simulink model "controlador_sugeno_obstaculos_velocidad"  (R2019a)
settings: Solver=FixedStepDiscrete  StartTime=0.0  StopTime=200  FixedStep=0.1  RelTol=1e-3
values from neighbouring files (symbols this model uses):
  arround_th = 0.01    [sugeno_obstaculos_velocidad.m]
  gain = 0.8    [sugeno_obstaculos_velocidad.m]
  offset_0 = -0.2    [sugeno_obstaculos_velocidad.m]
  offset_1 = -0.22    [sugeno_obstaculos_velocidad.m]
  offset_2 = -0.18    [sugeno_obstaculos_velocidad.m]
  offset_obs1 = 1.82    [sugeno_obstaculos_velocidad.m]
  offset_obs2 = -0.06    [sugeno_obstaculos_velocidad.m]
  saturation1_high = 1.27    [sugeno_obstaculos_velocidad.m]
  saturation1_high_lineal = 1.11    [sugeno_obstaculos_velocidad.m]
  saturation1_low = -1.39    [sugeno_obstaculos_velocidad.m]
  saturation1_low_lineal = -1.38    [sugeno_obstaculos_velocidad.m]
  saturation2_high = 4.53    [sugeno_obstaculos_velocidad.m]
  saturation2_high_lineal = 4.25    [sugeno_obstaculos_velocidad.m]
  saturation2_low = -4.47    [sugeno_obstaculos_velocidad.m]
  saturation2_low_lineal = -4.15    [sugeno_obstaculos_velocidad.m]
  saturation3_high = 3.31    [sugeno_obstaculos_velocidad.m]
  saturation3_high_lineal = 3.30    (= 3.3)    [sugeno_obstaculos_velocidad.m]
  saturation3_low = -2.01    [sugeno_obstaculos_velocidad.m]
  saturation3_low_lineal = -2    [sugeno_obstaculos_velocidad.m]
  saturation4_high = 2.37    [sugeno_obstaculos_velocidad.m]
  saturation4_high_lineal = 2.31    [sugeno_obstaculos_velocidad.m]
  saturation4_low = -5    [sugeno_obstaculos_velocidad.m]
  saturation4_low_lineal = -5    [sugeno_obstaculos_velocidad.m]
  saturation5_high = 4.71    [sugeno_obstaculos_velocidad.m]
  saturation5_high_lineal = 4.57    [sugeno_obstaculos_velocidad.m]
  saturation5_low = -3.57    [sugeno_obstaculos_velocidad.m]
  saturation5_low_lineal = -2.87    [sugeno_obstaculos_velocidad.m]
  Ts = 100e-3    (= 0.1)    [sugeno_obstaculos_velocidad.m]
undefined symbols (not defined in the file or in its folder): Angular, Linear
libraries: robotlib x11, fuzblock x2, robotcorelib x1
settings Model: EnablePacing=on  Creator=pizarro  LastModifiedBy=juanjosecordoba
settings DataIOCC: ReturnWorkspaceOutputs=off

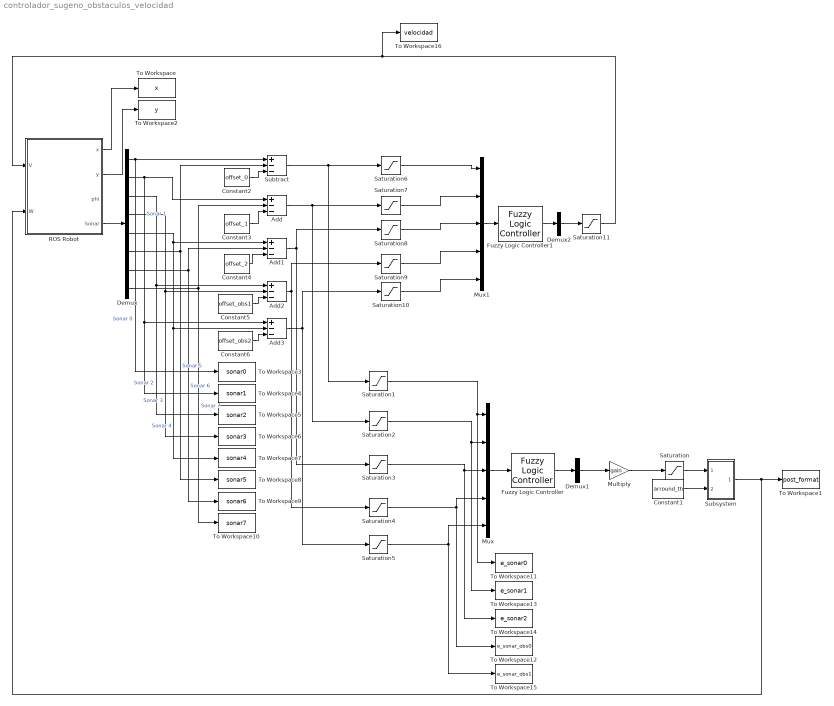
== system controlador_sugeno_obstaculos_velocidad ==
  Add{,1..3} (4 alike) : Sum  Inputs=+--
  Constant1 : Constant  Value=arround_th
  Constant2 : Constant  Value=offset_0  SampleTime=Ts
  Constant3 : Constant  Value=offset_1  SampleTime=Ts
  Constant4 : Constant  Value=offset_2  SampleTime=Ts
  Constant5 : Constant  Value=offset_obs1  SampleTime=Ts
  Constant6 : Constant  Value=offset_obs2  SampleTime=Ts
  Demux : Demux  Outputs=8
  Demux1 : Demux  Outputs=1
  Demux2 : Demux  Outputs=1
  Fuzzy Logic Controller : fuzblock/Fuzzy Logic  Controller  FIS=controller_name  OutputSampleNumber=101  DataType=double  FuzzifiedInputs=off  RuleFiringStrengths=off  RuleOutputs=off  AggregatedOutputs=off  SimulateUsing=Interpreted execution  OutOfRangeInputValueMessage=warning  NoRuleFiredMessage=warning  EmptyOutputFuzzySetMessage=warning
  Fuzzy Logic Controller1 : fuzblock/Fuzzy Logic  Controller  FIS=controller_name_lineal  OutputSampleNumber=101  DataType=double  FuzzifiedInputs=off  RuleFiringStrengths=off  RuleOutputs=off  AggregatedOutputs=off  SimulateUsing=Interpreted execution  OutOfRangeInputValueMessage=warning  NoRuleFiredMessage=warning  EmptyOutputFuzzySetMessage=warning
  Multiply : Gain  Gain=gain
  Mux : Mux  Inputs=5
  Mux1 : Mux  Inputs=5
  ROS Robot : Subsystem
  Saturation : Saturate  UpperLimit=pi  LowerLimit=-pi
  Saturation1 : Saturate  UpperLimit=saturation1_high  LowerLimit=saturation1_low
  Saturation10 : Saturate  UpperLimit=saturation5_high_lineal  LowerLimit=saturation5_low_lineal
  Saturation11 : Saturate  UpperLimit=1  LowerLimit=0
  Saturation2 : Saturate  UpperLimit=saturation2_high  LowerLimit=saturation2_low
  Saturation3 : Saturate  UpperLimit=saturation3_high  LowerLimit=saturation3_low
  Saturation4 : Saturate  UpperLimit=saturation4_high  LowerLimit=saturation4_low
  Saturation5 : Saturate  UpperLimit=saturation5_high  LowerLimit=saturation5_low
  Saturation6 : Saturate  UpperLimit=saturation1_high_lineal  LowerLimit=saturation1_low_lineal
  Saturation7 : Saturate  UpperLimit=saturation2_high_lineal  LowerLimit=saturation2_low_lineal
  Saturation8 : Saturate  UpperLimit=saturation3_high_lineal  LowerLimit=saturation3_low_lineal
  Saturation9 : Saturate  UpperLimit=saturation4_high_lineal  LowerLimit=saturation4_low_lineal
  Subsystem : Subsystem
  Subtract : Sum  Inputs=+--
  To Workspace : ToWorkspace  VariableName=x  SaveFormat=Structure With Time  SampleTime=Ts
  To Workspace1 : ToWorkspace  VariableName=post_format  SaveFormat=Structure With Time  SampleTime=Ts
  To Workspace10 : ToWorkspace  VariableName=sonar7  SaveFormat=Structure With Time  SampleTime=Ts
  To Workspace11 : ToWorkspace  VariableName=e_sonar0  SaveFormat=Structure With Time  SampleTime=Ts
  To Workspace12 : ToWorkspace  VariableName=e_sonar_obs0  SaveFormat=Structure With Time  SampleTime=Ts
  To Workspace13 : ToWorkspace  VariableName=e_sonar1  SaveFormat=Structure With Time  SampleTime=Ts
  To Workspace14 : ToWorkspace  VariableName=e_sonar2  SaveFormat=Structure With Time  SampleTime=Ts
  To Workspace15 : ToWorkspace  VariableName=e_sonar_obs1  SaveFormat=Structure With Time  SampleTime=Ts
  To Workspace16 : ToWorkspace  VariableName=velocidad  SaveFormat=Structure With Time  SampleTime=Ts
  To Workspace2 : ToWorkspace  VariableName=y  SaveFormat=Structure With Time  SampleTime=Ts
  To Workspace3 : ToWorkspace  VariableName=sonar0  SaveFormat=Structure With Time  SampleTime=Ts
  To Workspace4 : ToWorkspace  VariableName=sonar1  SaveFormat=Structure With Time  SampleTime=Ts
  To Workspace5 : ToWorkspace  VariableName=sonar2  SaveFormat=Structure With Time  SampleTime=Ts
  To Workspace6 : ToWorkspace  VariableName=sonar3  SaveFormat=Structure With Time  SampleTime=Ts
  To Workspace7 : ToWorkspace  VariableName=sonar4  SaveFormat=Structure With Time  SampleTime=Ts
  To Workspace8 : ToWorkspace  VariableName=sonar5  SaveFormat=Structure With Time  SampleTime=Ts
  To Workspace9 : ToWorkspace  VariableName=sonar6  SaveFormat=Structure With Time  SampleTime=Ts
  wires:
  ROS Robot/4(Sonar) -> Demux/1
  Fuzzy Logic Controller/1 -> Demux1/1
  Mux/1 -> Fuzzy Logic Controller/1
  Demux/1 -> Subtract/1, To Workspace3/1  "Sonar 0"
  Demux1/1 -> Multiply/1
  Saturation/1 -> Subsystem/1(value)
  Subsystem/1(Out1) -> ROS Robot/2(W), To Workspace1/1
  Constant1/1 -> Subsystem/2(arround_zero)
  Constant2/1 -> Subtract/3
  Constant3/1 -> Add/3
  Constant4/1 -> Add1/3
  Demux/2 -> Add3/1, To Workspace4/1, Add/1  "Sonar 1"
  Demux/6 -> Subtract/2, To Workspace8/1  "Sonar 5"
  Demux/5 -> Add3/2, To Workspace7/1, Add1/1  "Sonar 4"
  Demux/8 -> Add/2, To Workspace10/1  "Sonar 7"
  Demux/7 -> To Workspace9/1, Add1/2  "Sonar 6"
  Constant5/1 -> Add2/3
  Demux/3 -> To Workspace5/1, Add2/1  "Sonar 2"
  Demux/4 -> Add2/2, To Workspace6/1  "Sonar 3"
  Constant6/1 -> Add3/3
  ROS Robot/1(x) -> To Workspace/1
  ROS Robot/2(y) -> To Workspace2/1
  Subtract/1 -> Saturation6/1, Saturation1/1
  Add/1 -> Saturation7/1, Saturation2/1
  Add1/1 -> Saturation8/1, Saturation3/1
  Add2/1 -> Saturation9/1, Saturation4/1
  Add3/1 -> Saturation10/1, Saturation5/1
  Multiply/1 -> Saturation/1
  Saturation1/1 -> To Workspace11/1, Mux/1
  Saturation2/1 -> Mux/2, To Workspace13/1
  Saturation3/1 -> Mux/3, To Workspace14/1
  Saturation4/1 -> To Workspace12/1, Mux/4
  Saturation5/1 -> To Workspace15/1, Mux/5
  Saturation7/1 -> Mux1/2
  Saturation10/1 -> Mux1/5
  Saturation6/1 -> Mux1/1
  Saturation9/1 -> Mux1/4
  Saturation8/1 -> Mux1/3
  Mux1/1 -> Fuzzy Logic Controller1/1
  Fuzzy Logic Controller1/1 -> Demux2/1
  Demux2/1 -> Saturation11/1
  Saturation11/1 -> ROS Robot/1(V), To Workspace16/1

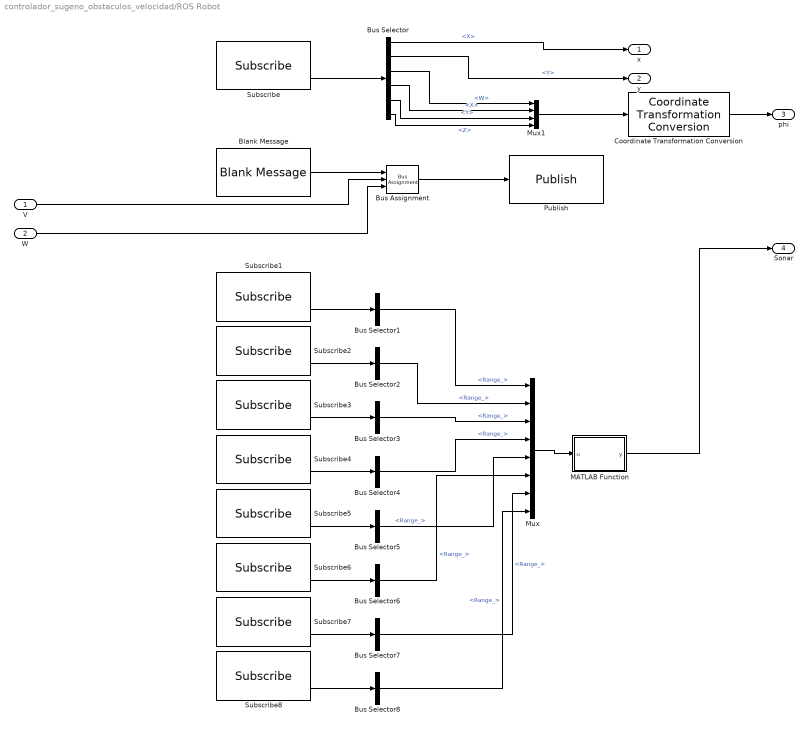
== system controlador_sugeno_obstaculos_velocidad/ROS Robot ==
  V : Inport
  W : Inport  Port=2
  Blank Message : robotlib/Blank Message  messageClass=Message  entityType=geometry_msgs/Twist  messageType=geometry_msgs/Twist  SampleTime=-1
      settings: SourceProductBaseCode=RO
  Bus Assignment : BusAssignment  AssignedSignals=Linear.X,Angular.Z
  Bus Selector : BusSelector  OutputSignals=Pose.Pose.Position.X,Pose.Pose.Position.Y,Pose.Pose.Orientation.W,Pose.Pose.Orientation.X,Pose.Pose.Orientation.Y,Pose.Pose.Orientation.Z
  Bus Selector{1..8} (8 alike) : BusSelector  OutputSignals=Range_
  Coordinate Transformation Conversion : robotcorelib/Coordinate Transformation Conversion  InputRepresentation=Quaternion  InputEulerSequence=ZYX  ShowTrVecInputPort=on  OutputRepresentation=Euler Angles  OutputEulerSequence=ZYX  ShowTrVecOutputPort=on  SimulateUsing=Interpreted execution
      settings: SourceProductBaseCode=RO
  MATLAB Function : MATLAB Function  TreatAsAtomicUnit=on
  Mux : Mux  Inputs=8
  Mux1 : Mux
  Publish : robotlib/Publish  topicSource=Select from ROS network  topic=/robot0/cmd_vel  messageType=geometry_msgs/Twist  messageQueueLength=1
      settings: SourceProductBaseCode=RO
  Subscribe : robotlib/Subscribe  topicSource=Select from ROS network  topic=/robot0/odom  messageType=nav_msgs/Odometry  sampleTime=-1  messageQueueLength=1
      settings: SourceProductBaseCode=RO
  Subscribe1 : robotlib/Subscribe  topicSource=Select from ROS network  topic=/robot0/sonar_0  messageType=sensor_msgs/Range  sampleTime=-1  messageQueueLength=1
      settings: SourceProductBaseCode=RO
  Subscribe2 : robotlib/Subscribe  topicSource=Select from ROS network  topic=/robot0/sonar_1  messageType=sensor_msgs/Range  sampleTime=-1  messageQueueLength=1
      settings: SourceProductBaseCode=RO
  Subscribe3 : robotlib/Subscribe  topicSource=Select from ROS network  topic=/robot0/sonar_2  messageType=sensor_msgs/Range  sampleTime=-1  messageQueueLength=1
      settings: SourceProductBaseCode=RO
  Subscribe4 : robotlib/Subscribe  topicSource=Select from ROS network  topic=/robot0/sonar_3  messageType=sensor_msgs/Range  sampleTime=-1  messageQueueLength=1
      settings: SourceProductBaseCode=RO
  Subscribe5 : robotlib/Subscribe  topicSource=Select from ROS network  topic=/robot0/sonar_4  messageType=sensor_msgs/Range  sampleTime=-1  messageQueueLength=1
      settings: SourceProductBaseCode=RO
  Subscribe6 : robotlib/Subscribe  topicSource=Select from ROS network  topic=/robot0/sonar_5  messageType=sensor_msgs/Range  sampleTime=-1  messageQueueLength=1
      settings: SourceProductBaseCode=RO
  Subscribe7 : robotlib/Subscribe  topicSource=Select from ROS network  topic=/robot0/sonar_6  messageType=sensor_msgs/Range  sampleTime=-1  messageQueueLength=1
      settings: SourceProductBaseCode=RO
  Subscribe8 : robotlib/Subscribe  topicSource=Select from ROS network  topic=/robot0/sonar_7  messageType=sensor_msgs/Range  sampleTime=-1  messageQueueLength=1
      settings: SourceProductBaseCode=RO
  x : Outport
  y : Outport  Port=2
  phi : Outport  Port=3
  Sonar : Outport  Port=4
  wires:
  Bus Selector/1 -> x/1  "<X>"
  Blank Message/1 -> Bus Assignment/1
  Subscribe/2 -> Bus Selector/1
  Bus Assignment/1 -> Publish/1
  Bus Selector/2 -> y/1  "<Y>"
  Subscribe1/2 -> Bus Selector1/1
  V/1 -> Bus Assignment/2
  W/1 -> Bus Assignment/3
  Subscribe2/2 -> Bus Selector2/1
  Subscribe3/2 -> Bus Selector3/1
  Subscribe5/2 -> Bus Selector5/1
  Subscribe4/2 -> Bus Selector4/1
  Subscribe6/2 -> Bus Selector6/1
  Subscribe7/2 -> Bus Selector7/1
  Bus Selector1/1 -> Mux/1  "<Range_>"
  Bus Selector2/1 -> Mux/2  "<Range_>"
  Bus Selector3/1 -> Mux/3  "<Range_>"
  Bus Selector4/1 -> Mux/4  "<Range_>"
  Bus Selector5/1 -> Mux/5  "<Range_>"
  Bus Selector6/1 -> Mux/6  "<Range_>"
  Bus Selector7/1 -> Mux/7  "<Range_>"
  Subscribe8/2 -> Bus Selector8/1
  Bus Selector8/1 -> Mux/8  "<Range_>"
  Bus Selector/3 -> Mux1/1  "<W>"
  Bus Selector/4 -> Mux1/2  "<X>"
  Bus Selector/5 -> Mux1/3  "<Y>"
  Bus Selector/6 -> Mux1/4  "<Z>"
  Mux1/1 -> Coordinate Transformation Conversion/1
  Coordinate Transformation Conversion/1 -> phi/1
  Mux/1 -> MATLAB Function/1(u)
  MATLAB Function/1(y) -> Sonar/1

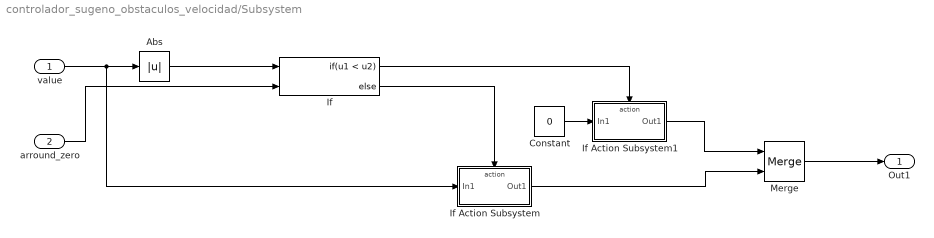
== system controlador_sugeno_obstaculos_velocidad/Subsystem ==
  value : Inport
  arround_zero : Inport  Port=2
  Abs : Abs
  Constant : Constant  Value=0  SampleTime=Ts
  If : If  NumInputs=2  IfExpression=u1 < u2
  If Action Subsystem : Subsystem  TreatAsAtomicUnit=on
  If Action Subsystem1 : Subsystem  TreatAsAtomicUnit=on
  Merge : Merge
  Out1 : Outport
  wires:
  If/1 -> If Action Subsystem1/Action
  If/2 -> If Action Subsystem/Action
  arround_zero/1 -> If/2
  If Action Subsystem1/1(Out1) -> Merge/1
  If Action Subsystem/1(Out1) -> Merge/2
  Merge/1 -> Out1/1
  value/1 -> Abs/1, If Action Subsystem/1(In1)
  Constant/1 -> If Action Subsystem1/1(In1)
  Abs/1 -> If/1

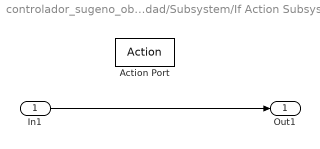
== system controlador_sugeno_obstaculos_velocidad/Subsystem/If Action Subsystem ==
  In1 : Inport
  Action Port : ActionPort  ActionPortLabel=else
  Out1 : Outport
  wires:
  In1/1 -> Out1/1

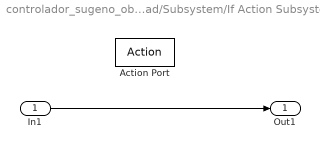
== system controlador_sugeno_obstaculos_velocidad/Subsystem/If Action Subsystem1 ==
  In1 : Inport
  Action Port : ActionPort  ActionPortLabel=if(u1 < u2)
  Out1 : Outport
  wires:
  In1/1 -> Out1/1

== matlab function controlador_sugeno_obstaculos_velocidad/ROS Robot/MATLAB Function ==
  data: u input; y output
function y = fcn(u)
u(isinf(u))=5.0;
y = u;
